simulink model "chap8_4sim"  (Simulink 5.0)
settings: Solver=ode45  StartTime=0.0  StopTime=2  FixedStep=0.001  RelTol=1e-3
settings Model: LastModifiedBy=Administrator  ExtModeTrigMode=oneshot  ExtModeArmWhenConnect=off  LimitDataPoints=off  BooleanDataType=off

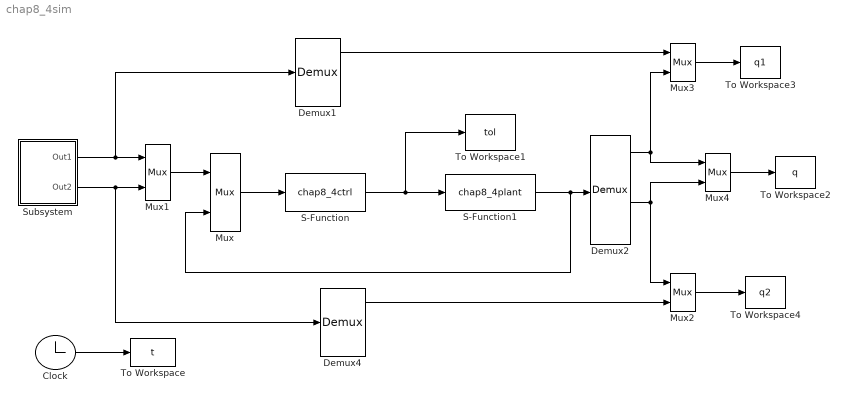
== system chap8_4sim ==
  Clock : Clock
      settings: Decimation=10
  Demux1 : Demux  Outputs=3
  Demux2 : Demux
  Demux4 : Demux  Outputs=3
  Mux{,1..4} (5 alike) : Mux  Inputs=2
  S-Function : S-Function  FunctionName=chap8_4ctrl
  S-Function1 : S-Function  FunctionName=chap8_4plant  Parameters=0.1,0.1
  Subsystem : Subsystem
  To Workspace : ToWorkspace  VariableName=t  SampleTime=-1  SaveFormat=Array
  To Workspace1 : ToWorkspace  VariableName=tol  SampleTime=-1  SaveFormat=Array
  To Workspace2 : ToWorkspace  VariableName=q  SampleTime=-1  SaveFormat=Array
  To Workspace3 : ToWorkspace  VariableName=q1  SampleTime=-1  SaveFormat=Array
  To Workspace4 : ToWorkspace  VariableName=q2  SampleTime=-1  SaveFormat=Array
  wires:
  Mux/1 -> S-Function/1
  Mux2/1 -> To Workspace4/1
  Mux3/1 -> To Workspace3/1
  S-Function/1 -> S-Function1/1, To Workspace1/1
  S-Function1/1 -> Mux/2, Demux2/1
  Demux2/3 -> Mux2/1, Mux4/2
  Mux1/1 -> Mux/1
  Demux4/1 -> Mux2/2
  Subsystem/1(Out1) -> Mux1/1, Demux1/1
  Subsystem/2(Out2) -> Mux1/2, Demux4/1
  Demux2/1 -> Mux3/2, Mux4/1
  Demux1/1 -> Mux3/1
  Clock/1 -> To Workspace/1
  Mux4/1 -> To Workspace2/1

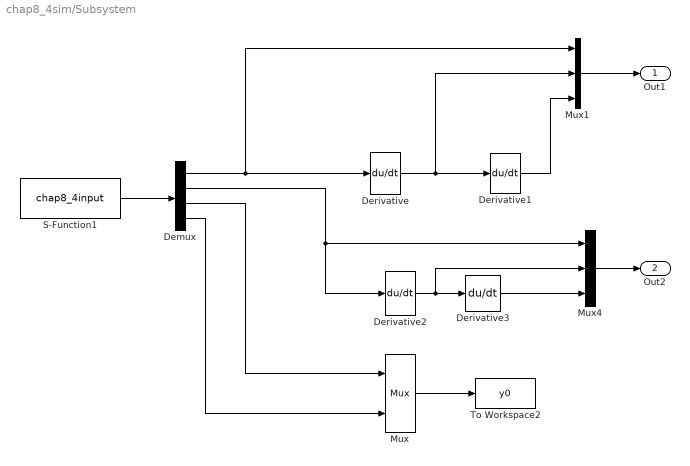
== system chap8_4sim/Subsystem ==
  Demux : Demux
  Derivative{,1..3} (4 alike) : Derivative
  Mux : Mux  Inputs=2
  Mux1 : Mux  Inputs=3
  Mux4 : Mux  Inputs=3
  S-Function1 : S-Function  FunctionName=chap8_4input
  To Workspace2 : ToWorkspace  VariableName=y0  SampleTime=-1  SaveFormat=Array
  Out1 : Outport
  Out2 : Outport  Port=2
  wires:
  S-Function1/1 -> Demux/1
  Derivative/1 -> Derivative1/1, Mux1/2
  Derivative1/1 -> Mux1/3
  Mux1/1 -> Out1/1
  Mux4/1 -> Out2/1
  Derivative2/1 -> Derivative3/1, Mux4/2
  Derivative3/1 -> Mux4/3
  Demux/1 -> Derivative/1, Mux1/1
  Demux/2 -> Derivative2/1, Mux4/1
  Demux/3 -> Mux/1
  Demux/4 -> Mux/2
  Mux/1 -> To Workspace2/1
